simulink model "benchmark"  (R2019b)
settings: Solver=ode45  StartTime=0.0  StopTime=14  FixedStep=0.01  RelTol=1e-5  AbsTol=1e-8
values from neighbouring files (symbols this model uses):
  carb1 = 0    [asm1init.m]
  carb2 = 0    [asm1init.m]
  carb3 = 0    [asm1init.m]
  carb4 = 0    [asm1init.m]
  carb5 = 0    [asm1init.m]
  DIM = [ area height ]    [settler1dinit.m]
  Kfeedforward = 0    [reginit.m]
  KLa1 = 0    [asm1init.m]
  KLa2 = 0    [asm1init.m]
  KLa3 = 240    [asm1init.m]
  KLa4 = 240    [asm1init.m]
  KLa5_max = 360    [sensorinit.m]
  KLa5offset = 144    [reginit.m]
  KQintr = 10000    [reginit.m]
  KSO5 = 25    [reginit.m]
  LAYER = [ feedlayer nooflayers ]    [settler1dinit.m]
  max_SNO2 = 20    [sensorinit.m]
  max_SO5 = 10    [sensorinit.m]
  min_SNO2 = 0    [sensorinit.m]
  min_SO5 = 0    [sensorinit.m]
  MODELTYPE = [ 0 ]    [settler1dinit.m]
  noiseseed_SNO2 = 2    [sensorinit.m]
  noiseseed_SO5 = 1    [sensorinit.m]
  noisesource_SNO2 = 1    [sensorinit.m]
  noisesource_SO5 = 1    [sensorinit.m]
  PAR1 = [ mu_H  K_S  K_OH  K_NO  b_H  mu_A  K_NH  K_OA  b_A  ny_g  k_a  k_h  K_X  ny_h  Y_H  Y_A  f_P  i_XB  i_XP X_I2TSS  X_S2TSS  X_BH2TSS  X_BA2TSS  X_P2TSS ]    [asm1init.m]
  PAR2 = PAR1    [asm1init.m]
  PAR3 = PAR1    [asm1init.m]
  PAR4 = PAR1    [asm1init.m]
  PAR5 = PAR1    [asm1init.m]
  Qffref = 3    [reginit.m]
  Qin0 = 18446    [asm1init.m]    (also in states.mat)
  Qintr = 3*Qin0    (= 55338)    [asm1init.m]    (also in savestatesdyn.m = Qintrreg(:,3); states.mat = 16194.6247784)
  Qintr_max = 5*Qin0    [sensorinit.m]
  Qintrawstate = 0    [reginit.m]    (also in states.mat)
  Qintrintstate = 0    [reginit.m]    (also in states.mat = -1584.65140052)
  Qintroffset = 18500    [reginit.m]
  QintrT = T*10    (= 0.001)    [asm1init.m]
  SETTLERINIT = [ TSS_1 TSS_2 TSS_3 TSS_4 TSS_5 TSS_6 TSS_7 TSS_8 TSS_9 TSS_10  SI_1 SI_2 SI_3 SI_4 SI_5 SI_6 SI_7 SI_8 SI_9 SI_10  SS_1 SS_2 SS_3 SS_4 SS_5 SS_6 SS_7 SS_8 SS_9 SS_10  SO_1 SO_2 SO_3 SO_4 SO_5 SO_6 SO_7 SO_8 SO_9 SO_10  SNO_1 SNO_2 SNO_3 SNO_4 SNO_5 SNO_6 SNO_7 SNO_8 SNO_9 SNO_10  SNH_1 SNH_2 SNH_3 SNH_4 SNH_5 SNH_6 SNH_7 SNH_8 SNH_9 SNH_10 SND_1 SND_2 SND_3 SND_4 SND_5 SND_6 SND_7 SND_8 SND_9 SND ...(+77 chars)    [savestatesdyn.m]    (also in settler1dinit.m; states.mat = [12.59234379 18.2836278135 29.6255352805 68.5613149178 351.4)
  SETTLERPAR = [ v0_max v0 r_h r_p f_ns X_t ]    [settler1dinit.m]
  SNO2ref = 1    [reginit.m]
  SO5awstate = 0    [reginit.m]    (also in states.mat = 333.995683123)
  SO5intstate = 0    [reginit.m]    (also in states.mat = -324.385367613)
  SO5ref = 2    [reginit.m]
  SOSAT1 = 8    [asm1init.m]
  SOSAT2 = SOSAT1    (= 8)    [asm1init.m]
  SOSAT3 = SOSAT1    (= 8)    [asm1init.m]
  SOSAT4 = SOSAT1    (= 8)    [asm1init.m]
  SOSAT5 = SOSAT1    (= 8)    [asm1init.m]
  std_SNO2 = 0.025    [sensorinit.m]
  std_SO5 = 0.025    [sensorinit.m]
  T = 0.0001    [asm1init.m]
  T_KLa5 = T90_KLa5/(24*60)/3.89    (= 0.000714081690945)    [sensorinit.m]
  T_SNO2 = T90_SNO2/(24*60)/11.7724    (= 0.000589891988417)    [sensorinit.m]
  T_SO5 = T90_SO5/(24*60)/3.89    (= 0.000178520422736)    [sensorinit.m]
  TiQintr = 0.025    [reginit.m]
  TiSO5 = 0.002    [reginit.m]
  TtQintr = 0.015    [reginit.m]
  TtSO5 = 0.001    [reginit.m]
  useantiwindupQintr = 1    [reginit.m]
  useantiwindupSO5 = 1    [reginit.m]
  useideal_KLa5 = 0    [sensorinit.m]
  useideal_SNO2 = 0    [sensorinit.m]
  useideal_SO5 = 0    [sensorinit.m]
  usenoise_SNO2 = 1    [sensorinit.m]
  usenoise_SO5 = 1    [sensorinit.m]
  VOL1 = 1000    [asm1init.m]
  VOL2 = VOL1    (= 1000)    [asm1init.m]
  VOL3 = 1333    [asm1init.m]
  VOL4 = VOL3    (= 1333)    [asm1init.m]
  VOL5 = VOL3    (= 1333)    [asm1init.m]
  XINIT1 = XINIT1.*(rand(1, 15)/2)    [asm1init.m]    (also in savestatesdyn.m = [ S_I1  S_S1  X_I1  X_S1  X_BH1  X_BA1  X_P1  S_O1  S_NO1  S; states.mat = [30 3.19850453028 1132.76234619 97.3159244857 2519.85046875 )
  XINIT2 = XINIT2.*(rand(1, 15)/2)    [asm1init.m]    (also in savestatesdyn.m = [ S_I2  S_S2  X_I2  X_S2  X_BH2  X_BA2  X_P2  S_O2  S_NO2  S; states.mat = [30 1.66685060474 1124.48673742 89.8629588992 2501.10529682 )
  XINIT3 = XINIT3.*(rand(1, 15)/2)    [asm1init.m]    (also in savestatesdyn.m = [ S_I3  S_S3  X_I3  X_S3  X_BH3  X_BA3  X_P3  S_O3  S_NO3  S; states.mat = [30 1.21920729218 1120.83917563 67.9873482569 2499.89769316 )
  XINIT4 = XINIT4.*(rand(1, 15)/2)    [asm1init.m]    (also in savestatesdyn.m = [ S_I4  S_S4  X_I4  X_S4  X_BH4  X_BA4  X_P4  S_O4  S_NO4  S; states.mat = [30 0.970059599738 1121.87647389 52.9944958383 2504.40148464)
  XINIT5 = XINIT5.*(rand(1, 15)/2)    [asm1init.m]    (also in savestatesdyn.m = [ S_I5  S_S5  X_I5  X_S5  X_BH5  X_BA5  X_P5  S_O5  S_NO5  S; states.mat = [30 0.802872668211 1124.31099208 43.2311724286 2508.27851004)
  XINITDELAY = [ S_I_ASin  S_S_ASin  X_I_ASin  X_S_ASin  X_BH_ASin  X_BA_ASin  X_P_ASin  S_O_ASin  S_NO_ASin  S_NH_ASin  S_ND_ASin  X_ND_ASin  S_ALK_ASin TSS_ASin Q_ASin ]    [asm1init.m]    (also in savestatesdyn.m; states.mat = [1591648.02176 1269347.74818 60483506.753 5993584.75542 1336)
settings Model: ExtModeTrigMode=oneshot  ExtModeArmWhenConnect=off  ExtModeAutoUpdateStatusClock=off  Creator=ielulf  LastModifiedBy=ielsaagi
settings SolverCC: AutoScaleAbsTol=off
settings DataIOCC: SaveFormat=Array  SignalLoggingSaveFormat=ModelDataLogs  SaveOutput=off  ReturnWorkspaceOutputs=off  TimeSaveName=t  SignalLoggingName=sigsOut  OutputOption=SpecifiedOutputTimes  OutputTimes=[7:(1/96):14]
settings OptimizationCC: BlockReduction=off  BooleanDataType=off  InitFltsAndDblsToZero=on  LifeSpan=inf
settings DebuggingCC: AlgebraicLoopMsg=none  SaveWithParameterizedLinksMsg=none  UnderspecifiedInitializationDetection=Classic  MergeDetectMultiDrivingBlocksExec=none  SignalResolutionControl=TryResolveAllWithWarning  InheritedTsInSrcMsg=none  MultiTaskDSMMsg=warning  MultiTaskCondExecSysMsg=none  FcnCallInpInsideContextMsg=warning  UnconnectedOutputMsg=none  SFUnexpectedBacktrackingDiag=warning  SFNoUnconditionalDefaultTransitionDiag=warning  SFExecutionAtInitializationDiag=none  ArithmeticOperatorsInVariantConditions=warning
settings HardwareCC: ProdBitPerPointer=32  ProdBitPerSizeT=32  ProdBitPerPtrDiffT=32  ProdLargestAtomicFloat=None  ProdIntDivRoundTo=Undefined  ProdEndianess=Unspecified  ProdWordSize=32  ProdHWDeviceType=32-bit Generic  TargetUnknown=on
settings ModelReferenceCC: PropagateSignalLabelsOutOfModel=off
settings RTWCC: TemplateMakefile=grt_unix.tmf
settings CodeAppCC: StateflowObjectComments=on
settings GRTTargetCC: TargetFcnLib=ansi_tfl_tmw.mat  TargetLangStandard=C89/C90 (ANSI)  CombineOutputUpdateFcns=off  GRTInterface=on
settings ConfigComp: CovMetricSettings=dw  CovHtmlReporting=on  CovSaveCumulativeToWorkspaceVar=on  CovSaveSingleToWorkspaceVar=on

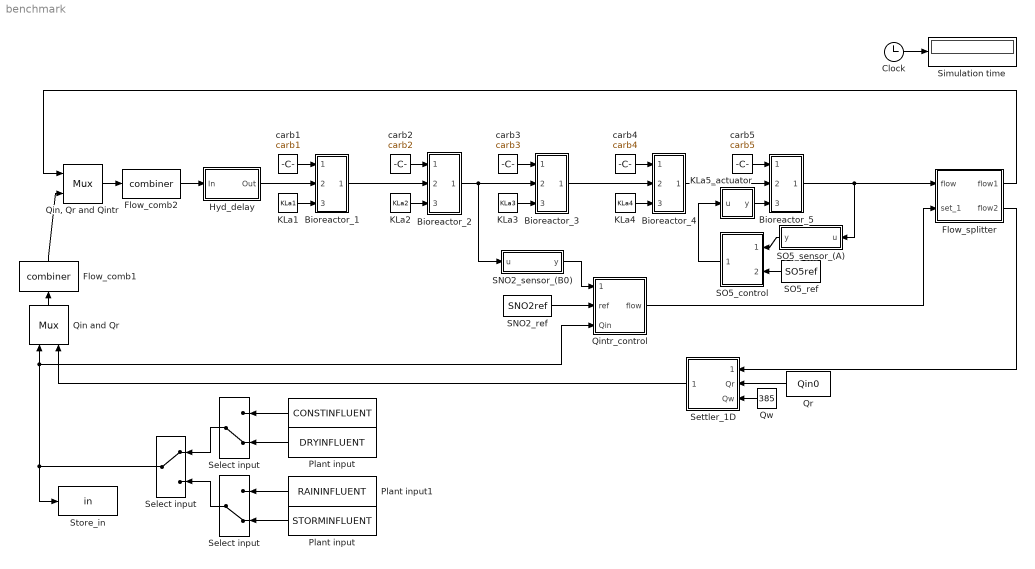
== system benchmark ==
  " " : FromWorkspace  VariableName=CONSTINFLUENT  OutputAfterFinalValue=Holding final value
  " Select input" : ManualSwitch
  Bioreactor_1 : Subsystem
  Bioreactor_2 : Subsystem
  Bioreactor_3 : Subsystem
  Bioreactor_4 : Subsystem
  Bioreactor_5 : Subsystem
  Clock : Clock
  Flow_comb1 : S-Function  FunctionName=combiner  SFunctionDeploymentMode=off  EnableBusSupport=off
  Flow_comb2 : S-Function  FunctionName=combiner  SFunctionDeploymentMode=off  EnableBusSupport=off
  Flow_splitter : Subsystem
  Hyd_delay : Subsystem
  KLa1 : Constant  Value=KLa1
  KLa2 : Constant  Value=KLa2
  KLa3 : Constant  Value=KLa3
  KLa4 : Constant  Value=KLa4
  KLa5_actuator : Subsystem
  Plant input : FromWorkspace  VariableName=DRYINFLUENT  OutputAfterFinalValue=Holding final value
  "Plant input " : FromWorkspace  VariableName=STORMINFLUENT  OutputAfterFinalValue=Holding final value
  Plant input1 : FromWorkspace  VariableName=RAININFLUENT  OutputAfterFinalValue=Holding final value
  Qin and Qr : Mux  Inputs=2
  "Qin, Qr and Qintr" : Mux  Inputs=2
  Qintr_control : Subsystem
  Qr : Constant  Value=Qin0
  Qw : Constant  Value=385
  SNO2_ref : Constant  Value=SNO2ref
  SNO2_sensor_(B0) : Subsystem
  SO5_control : Subsystem
  SO5_ref : Constant  Value=SO5ref
  SO5_sensor_(A) : Subsystem
  Select input : ManualSwitch  CurrentSetting=0
  "Select input " : ManualSwitch  CurrentSetting=0
  Settler_1D : Subsystem
  Simulation time : Display
  Store_in : ToWorkspace  VariableName=in  SampleTime=-1
  carb1 : Constant  Value=carb1
  carb2 : Constant  Value=carb2
  carb3 : Constant  Value=carb3
  carb4 : Constant  Value=carb4
  carb5 : Constant  Value=carb5
  wires:
  Qin and Qr/1 -> Flow_comb1/1
  Flow_comb1/1 -> "Qin, Qr and Qintr"/2
  "Qin, Qr and Qintr"/1 -> Flow_comb2/1
  Flow_splitter/1(flow1) -> "Qin, Qr and Qintr"/1
  Settler_1D/1(output) -> Qin and Qr/2
  Qw/1 -> Settler_1D/3(Qw)
  Flow_splitter/2(flow2) -> Settler_1D/1(feed)
  Qr/1 -> Settler_1D/2(Qr)
  Bioreactor_5/1(out) -> Flow_splitter/1(flow), SO5_sensor_(A)/1(u)
  Flow_comb2/1 -> Hyd_delay/1(In)
  Clock/1 -> Simulation time/1
  Plant input/1 -> Select input/2
  " "/1 -> Select input/1
  Hyd_delay/1(Out) -> Bioreactor_1/2(in)
  carb1/1 -> Bioreactor_1/1(carb)
  KLa1/1 -> Bioreactor_1/3(KLa)
  Bioreactor_1/1(out) -> Bioreactor_2/2(in)
  KLa2/1 -> Bioreactor_2/3(KLa)
  carb2/1 -> Bioreactor_2/1(carb)
  Bioreactor_2/1(out) -> Bioreactor_3/2(in), SNO2_sensor_(B0)/1(u)
  KLa3/1 -> Bioreactor_3/3(KLa)
  carb3/1 -> Bioreactor_3/1(carb)
  Bioreactor_3/1(out) -> Bioreactor_4/2(in)
  KLa4/1 -> Bioreactor_4/3(KLa)
  carb4/1 -> Bioreactor_4/1(carb)
  Bioreactor_4/1(out) -> Bioreactor_5/2(in)
  carb5/1 -> Bioreactor_5/1(carb)
  Plant input1/1 -> "Select input "/1
  "Plant input "/1 -> "Select input "/2
  Select input/1 -> " Select input"/1
  "Select input "/1 -> " Select input"/2
  " Select input"/1 -> Store_in/1, Qin and Qr/1, Qintr_control/3(Qin)
  SNO2_ref/1 -> Qintr_control/2(ref)
  SNO2_sensor_(B0)/1(y) -> Qintr_control/1(meas)
  Qintr_control/1(flow) -> Flow_splitter/2(set_1)
  SO5_ref/1 -> SO5_control/2(O2_ref)
  KLa5_actuator/1(y) -> Bioreactor_5/3(KLa)
  SO5_control/1(KLa) -> KLa5_actuator/1(u)
  SO5_sensor_(A)/1(y) -> SO5_control/1(O2_meas)

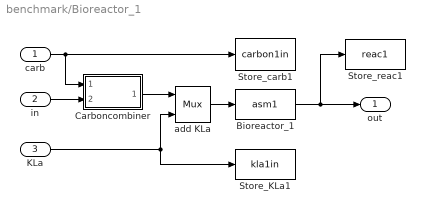
== system benchmark/Bioreactor_1 ==
  carb : Inport
  in : Inport  Port=2
  KLa : Inport  Port=3
  Bioreactor_1 : S-Function  FunctionName=asm1  Parameters=XINIT1,PAR1,VOL1,SOSAT1  SFunctionDeploymentMode=off  EnableBusSupport=off
  Carboncombiner : Subsystem
  Store_KLa1 : ToWorkspace  VariableName=kla1in  SampleTime=-1
  Store_carb1 : ToWorkspace  VariableName=carbon1in  SampleTime=-1
  Store_reac1 : ToWorkspace  VariableName=reac1  SampleTime=-1
  add KLa : Mux  Inputs=2
  out : Outport
  wires:
  add KLa/1 -> Bioreactor_1/1
  Bioreactor_1/1 -> out/1, Store_reac1/1
  Carboncombiner/1(Output) -> add KLa/1
  carb/1 -> Store_carb1/1, Carboncombiner/1(C_flow)
  in/1 -> Carboncombiner/2(Input)
  KLa/1 -> add KLa/2, Store_KLa1/1

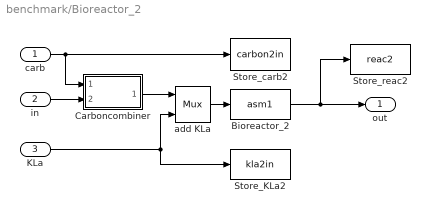
== system benchmark/Bioreactor_2 ==
  carb : Inport
  in : Inport  Port=2
  KLa : Inport  Port=3
  Bioreactor_2 : S-Function  FunctionName=asm1  Parameters=XINIT2,PAR2,VOL2,SOSAT2  SFunctionDeploymentMode=off  EnableBusSupport=off
  Carboncombiner : Subsystem
  Store_KLa2 : ToWorkspace  VariableName=kla2in  SampleTime=-1
  Store_carb2 : ToWorkspace  VariableName=carbon2in  SampleTime=-1
  Store_reac2 : ToWorkspace  VariableName=reac2  SampleTime=-1
  add KLa : Mux  Inputs=2
  out : Outport
  wires:
  Bioreactor_2/1 -> out/1, Store_reac2/1
  add KLa/1 -> Bioreactor_2/1
  Carboncombiner/1(Output) -> add KLa/1
  carb/1 -> Carboncombiner/1(C_flow), Store_carb2/1
  in/1 -> Carboncombiner/2(Input)
  KLa/1 -> add KLa/2, Store_KLa2/1

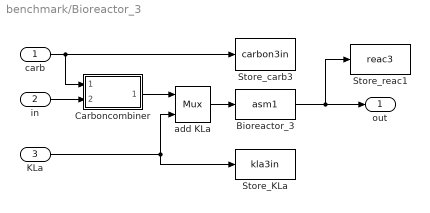
== system benchmark/Bioreactor_3 ==
  carb : Inport
  in : Inport  Port=2
  KLa : Inport  Port=3
  Bioreactor_3 : S-Function  FunctionName=asm1  Parameters=XINIT3,PAR3,VOL3,SOSAT3  SFunctionDeploymentMode=off  EnableBusSupport=off
  Carboncombiner : Subsystem
  Store_KLa : ToWorkspace  VariableName=kla3in  SampleTime=-1
  Store_carb3 : ToWorkspace  VariableName=carbon3in  SampleTime=-1
  Store_reac1 : ToWorkspace  VariableName=reac3  SampleTime=-1
  add KLa : Mux  Inputs=2
  out : Outport
  wires:
  Bioreactor_3/1 -> out/1, Store_reac1/1
  add KLa/1 -> Bioreactor_3/1
  Carboncombiner/1(Output) -> add KLa/1
  carb/1 -> Carboncombiner/1(C_flow), Store_carb3/1
  in/1 -> Carboncombiner/2(Input)
  KLa/1 -> add KLa/2, Store_KLa/1

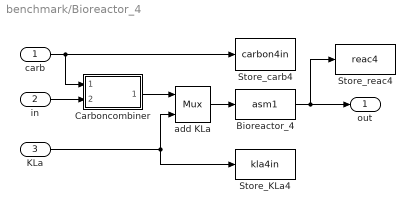
== system benchmark/Bioreactor_4 ==
  carb : Inport
  in : Inport  Port=2
  KLa : Inport  Port=3
  Bioreactor_4 : S-Function  FunctionName=asm1  Parameters=XINIT4,PAR4,VOL4,SOSAT4  SFunctionDeploymentMode=off  EnableBusSupport=off
  Carboncombiner : Subsystem
  Store_KLa4 : ToWorkspace  VariableName=kla4in  SampleTime=-1
  Store_carb4 : ToWorkspace  VariableName=carbon4in  SampleTime=-1
  Store_reac4 : ToWorkspace  VariableName=reac4  SampleTime=-1
  add KLa : Mux  Inputs=2
  out : Outport
  wires:
  Bioreactor_4/1 -> out/1, Store_reac4/1
  add KLa/1 -> Bioreactor_4/1
  Carboncombiner/1(Output) -> add KLa/1
  carb/1 -> Carboncombiner/1(C_flow), Store_carb4/1
  in/1 -> Carboncombiner/2(Input)
  KLa/1 -> add KLa/2, Store_KLa4/1

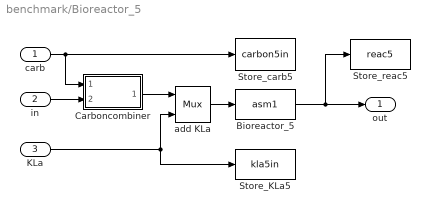
== system benchmark/Bioreactor_5 ==
  carb : Inport
  in : Inport  Port=2
  KLa : Inport  Port=3
  Bioreactor_5 : S-Function  FunctionName=asm1  Parameters=XINIT5,PAR5,VOL5,SOSAT5  SFunctionDeploymentMode=off  EnableBusSupport=off
  Carboncombiner : Subsystem
  Store_KLa5 : ToWorkspace  VariableName=kla5in  SampleTime=-1
  Store_carb5 : ToWorkspace  VariableName=carbon5in  SampleTime=-1
  Store_reac5 : ToWorkspace  VariableName=reac5  SampleTime=-1
  add KLa : Mux  Inputs=2
  out : Outport
  wires:
  Bioreactor_5/1 -> out/1, Store_reac5/1
  add KLa/1 -> Bioreactor_5/1
  Carboncombiner/1(Output) -> add KLa/1
  carb/1 -> Carboncombiner/1(C_flow), Store_carb5/1
  in/1 -> Carboncombiner/2(Input)
  KLa/1 -> add KLa/2, Store_KLa5/1

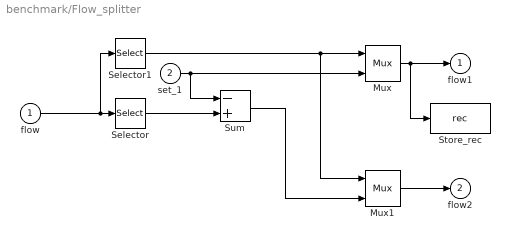
== system benchmark/Flow_splitter ==
  flow : Inport
  set_1 : Inport  Port=2
  Mux : Mux  Inputs=2
  Mux1 : Mux  Inputs=2
  Selector : Selector  InputPortWidth=15  IndexOptions=Index vector (dialog)  Indices=[15]  OutputSizes=1
  Selector1 : Selector  InputPortWidth=15  IndexOptions=Index vector (dialog)  Indices=[1 2 3 4 5 6 7 8 9 10 11 12 13 14]  OutputSizes=1
  Store_rec : ToWorkspace  VariableName=rec  SampleTime=-1
  Sum : Sum  Inputs=-+  SaturateOnIntegerOverflow=on  InputSameDT=on  OutDataTypeStr=Inherit: Same as first input
  flow1 : Outport
  flow2 : Outport  Port=2
  wires:
  flow/1 -> Selector1/1, Selector/1
  Mux/1 -> flow1/1, Store_rec/1
  Mux1/1 -> flow2/1
  set_1/1 -> Mux/2, Sum/1
  Selector/1 -> Sum/2
  Sum/1 -> Mux1/2
  Selector1/1 -> Mux/1, Mux1/1

== system benchmark/Hyd_delay ==
  In : Inport
  Demux : Demux  Outputs=[14,1]
  Hyd_delay : S-Function  FunctionName=hyddelayv3  Parameters=XINITDELAY,PAR1,T  SFunctionDeploymentMode=off  EnableBusSupport=off
  Mux : Mux  Inputs=2
  Product : Product  SaturateOnIntegerOverflow=on  OutDataTypeStr=Inherit: Same as first input
  Store_ASinput : ToWorkspace  VariableName=ASinput  SampleTime=-1
  Out : Outport
  wires:
  In/1 -> Hyd_delay/1
  Hyd_delay/1 -> Out/1, Demux/1
  Demux/1 -> Product/1
  Demux/2 -> Product/2, Mux/2
  Product/1 -> Mux/1
  Mux/1 -> Store_ASinput/1

== system benchmark/KLa5_actuator ==
  u : Inport
  Constant2 : Constant  Value=useideal_KLa5
  KLa5_actuator : TransferFcn  Denominator=[ T_KLa5*T_KLa5, 2*T_KLa5, 1]
  Switch1 : Switch  Threshold=0.5
  y : Outport
  wires:
  u/1 -> KLa5_actuator/1, Switch1/1
  Switch1/1 -> y/1
  KLa5_actuator/1 -> Switch1/3
  Constant2/1 -> Switch1/2

== system benchmark/Qintr_control ==
  meas : Inport
  ref : Inport  Port=2
  Qin : Inport  Port=3
  Selector : Selector  InputPortWidth=15  IndexOptions=Index vector (dialog)  Indices=[15]  OutputSizes=1
  Sum : Sum  Inputs=-+  SaturateOnIntegerOverflow=on  InputSameDT=on  OutDataTypeStr=Inherit: Same as first input
  cont_PI2 : Subsystem
  flow : Outport
  wires:
  meas/1 -> Sum/1
  Sum/1 -> cont_PI2/1(Error)
  cont_PI2/1(Out) -> flow/1
  Qin/1 -> Selector/1
  ref/1 -> Sum/2, cont_PI2/2(SNOref)
  Selector/1 -> cont_PI2/3(Qin)

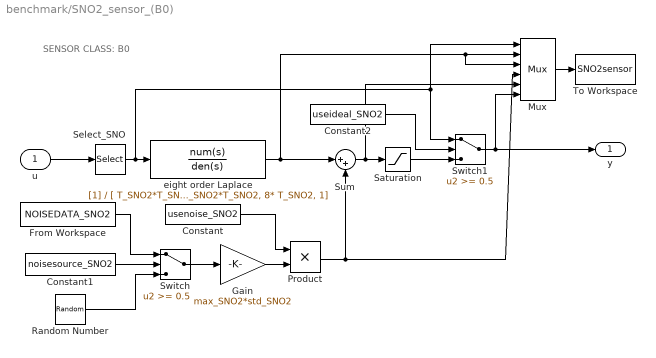
== system benchmark/SNO2_sensor_(B0) ==
  note: SENSOR CLASS: B0
  u : Inport
  Constant : Constant  Value=usenoise_SNO2
  Constant1 : Constant  Value=noisesource_SNO2
  Constant2 : Constant  Value=useideal_SNO2
  From Workspace : FromWorkspace  VariableName=NOISEDATA_SNO2  SampleTime=0
  Gain : Gain  Gain=max_SNO2*std_SNO2  SaturateOnIntegerOverflow=on  OutDataTypeStr=Inherit: Same as input  ParamDataTypeStr=Inherit: Same as input
  Mux : Mux  Inputs=6
  Product : Product  SaturateOnIntegerOverflow=on  InputSameDT=on  OutDataTypeStr=Inherit: Same as first input
  Random Number : RandomNumber  Seed=noiseseed_SNO2  SampleTime=1/1440
  Saturation : Saturate  UpperLimit=max_SNO2  LowerLimit=min_SNO2
  Select_SNO : Selector  InputPortWidth=15  IndexOptions=Index vector (dialog)  Indices=[9]  OutputSizes=1
  Sum : Sum  Inputs=|++  SaturateOnIntegerOverflow=on  InputSameDT=on  OutDataTypeStr=Inherit: Same as first input
  Switch : Switch  Threshold=0.5
  Switch1 : Switch  Threshold=0.5
  To Workspace : ToWorkspace  VariableName=SNO2sensor  SampleTime=-1
  eight order Laplace : TransferFcn  Denominator=[ T_SNO2*T_SNO2*T_SNO2*T_SNO2*T_SNO2*T_SNO2*T_SNO2*T_SNO2, 8*T_SNO2*T_SNO2*T_SNO2*T_SNO2*T_SNO2*T_SNO2*T_SNO2, 28*T_SNO2*T_SNO2*T_SNO2*T_SNO2*T_SNO2*T_SNO2, 56*T_SNO2*T_SNO2*T_SNO2*T_SNO2*T_SNO2, 70*T_SNO2*T_SNO2*T_SNO2*T_SNO2, 56*T_SNO2*T_SNO2*T_SNO2, 28*T_SNO2*T_SNO2, 8* T_SNO2, 1]
  y : Outport
  wires:
  Mux/1 -> To Workspace/1
  Constant2/1 -> Switch1/2
  Switch1/1 -> Mux/6, y/1
  Saturation/1 -> Switch1/3
  Random Number/1 -> Switch/3
  Constant1/1 -> Switch/2
  From Workspace/1 -> Switch/1
  Constant/1 -> Product/1
  Switch/1 -> Gain/1
  Gain/1 -> Product/2
  Select_SNO/1 -> Mux/1, Switch1/1, eight order Laplace/1
  u/1 -> Select_SNO/1
  Product/1 -> Mux/4, Sum/2
  eight order Laplace/1 -> Mux/3, Mux/2, Sum/1
  Sum/1 -> Mux/5, Saturation/1

== system benchmark/SO5_control ==
  O2_meas : Inport
  O2_ref : Inport  Port=2
  Sum : Sum  Inputs=-+  SaturateOnIntegerOverflow=on  InputSameDT=on  OutDataTypeStr=Inherit: Same as first input
  cont_PI : Subsystem
  KLa : Outport
  wires:
  Sum/1 -> cont_PI/1(In)
  O2_ref/1 -> Sum/2
  cont_PI/1(Out) -> KLa/1
  O2_meas/1 -> Sum/1

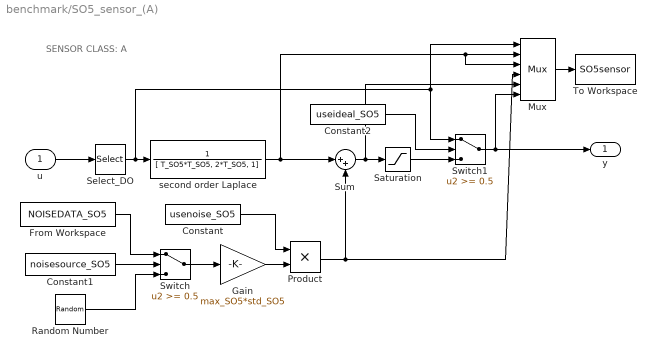
== system benchmark/SO5_sensor_(A) ==
  note: SENSOR CLASS: A
  u : Inport
  Constant : Constant  Value=usenoise_SO5
  Constant1 : Constant  Value=noisesource_SO5
  Constant2 : Constant  Value=useideal_SO5
  From Workspace : FromWorkspace  VariableName=NOISEDATA_SO5  SampleTime=0
  Gain : Gain  Gain=max_SO5*std_SO5  SaturateOnIntegerOverflow=on  OutDataTypeStr=Inherit: Same as input  ParamDataTypeStr=Inherit: Same as input
  Mux : Mux  Inputs=6
  Product : Product  SaturateOnIntegerOverflow=on  InputSameDT=on  OutDataTypeStr=Inherit: Same as first input
  Random Number : RandomNumber  Seed=noiseseed_SO5  SampleTime=1/1440
  Saturation : Saturate  UpperLimit=max_SO5  LowerLimit=min_SO5
  Select_DO : Selector  InputPortWidth=15  IndexOptions=Index vector (dialog)  Indices=[8]  OutputSizes=1
  Sum : Sum  Inputs=|++  SaturateOnIntegerOverflow=on  InputSameDT=on  OutDataTypeStr=Inherit: Same as first input
  Switch : Switch  Threshold=0.5
  Switch1 : Switch  Threshold=0.5
  To Workspace : ToWorkspace  VariableName=SO5sensor  SampleTime=-1
  second order Laplace : TransferFcn  Denominator=[ T_SO5*T_SO5, 2*T_SO5, 1]
  y : Outport
  wires:
  Mux/1 -> To Workspace/1
  Constant2/1 -> Switch1/2
  Switch1/1 -> Mux/6, y/1
  Saturation/1 -> Switch1/3
  Random Number/1 -> Switch/3
  Constant1/1 -> Switch/2
  From Workspace/1 -> Switch/1
  Constant/1 -> Product/1
  Switch/1 -> Gain/1
  Gain/1 -> Product/2
  Select_DO/1 -> Mux/1, Switch1/1, second order Laplace/1
  u/1 -> Select_DO/1
  Product/1 -> Mux/4, Sum/2
  second order Laplace/1 -> Mux/3, Mux/2, Sum/1
  Sum/1 -> Mux/5, Saturation/1

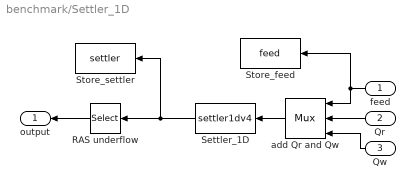
== system benchmark/Settler_1D ==
  feed : Inport
  Qr : Inport  Port=2
  Qw : Inport  Port=3
  RAS underflow : Selector  InputPortWidth=113  IndexOptions=Index vector (dialog)  Indices=[1 2 3 4 5 6 7 8 9 10 11 12 13 14 15]  OutputSizes=1
  Settler_1D : S-Function  FunctionName=settler1dv4  Parameters=SETTLERINIT,SETTLERPAR,DIM,LAYER,MODELTYPE  SFunctionDeploymentMode=off  EnableBusSupport=off
  Store_feed : ToWorkspace  VariableName=feed  SampleTime=-1
  Store_settler : ToWorkspace  VariableName=settler  SampleTime=-1
  add Qr and Qw : Mux  Inputs=3
  output : Outport
  wires:
  add Qr and Qw/1 -> Settler_1D/1
  Qr/1 -> add Qr and Qw/2
  Qw/1 -> add Qr and Qw/3
  feed/1 -> add Qr and Qw/1, Store_feed/1
  RAS underflow/1 -> output/1
  Settler_1D/1 -> RAS underflow/1, Store_settler/1

== system benchmark/Bioreactor_1/Carboncombiner ==
  C_flow : Inport
  Input : Inport  Port=2
  Carboncombiner : S-Function  FunctionName=carboncombiner  Parameters=CARBONSOURCECONC  SFunctionDeploymentMode=off  EnableBusSupport=off
  Mux : Mux  Inputs=2
  Output : Outport
  wires:
  C_flow/1 -> Mux/1
  Mux/1 -> Carboncombiner/1
  Carboncombiner/1 -> Output/1
  Input/1 -> Mux/2

== system benchmark/Bioreactor_2/Carboncombiner ==
  C_flow : Inport
  Input : Inport  Port=2
  Carboncombiner : S-Function  FunctionName=carboncombiner  Parameters=CARBONSOURCECONC  SFunctionDeploymentMode=off  EnableBusSupport=off
  Mux : Mux  Inputs=2
  Output : Outport
  wires:
  Input/1 -> Mux/2
  Carboncombiner/1 -> Output/1
  Mux/1 -> Carboncombiner/1
  C_flow/1 -> Mux/1

== system benchmark/Bioreactor_3/Carboncombiner ==
  C_flow : Inport
  Input : Inport  Port=2
  Carboncombiner : S-Function  FunctionName=carboncombiner  Parameters=CARBONSOURCECONC  SFunctionDeploymentMode=off  EnableBusSupport=off
  Mux : Mux  Inputs=2
  Output : Outport
  wires:
  Input/1 -> Mux/2
  Carboncombiner/1 -> Output/1
  Mux/1 -> Carboncombiner/1
  C_flow/1 -> Mux/1

== system benchmark/Bioreactor_4/Carboncombiner ==
  C_flow : Inport
  Input : Inport  Port=2
  Carboncombiner : S-Function  FunctionName=carboncombiner  Parameters=CARBONSOURCECONC  SFunctionDeploymentMode=off  EnableBusSupport=off
  Mux : Mux  Inputs=2
  Output : Outport
  wires:
  Input/1 -> Mux/2
  Carboncombiner/1 -> Output/1
  Mux/1 -> Carboncombiner/1
  C_flow/1 -> Mux/1

== system benchmark/Bioreactor_5/Carboncombiner ==
  C_flow : Inport
  Input : Inport  Port=2
  Carboncombiner : S-Function  FunctionName=carboncombiner  Parameters=CARBONSOURCECONC  SFunctionDeploymentMode=off  EnableBusSupport=off
  Mux : Mux  Inputs=2
  Output : Outport
  wires:
  Input/1 -> Mux/2
  Carboncombiner/1 -> Output/1
  Mux/1 -> Carboncombiner/1
  C_flow/1 -> Mux/1

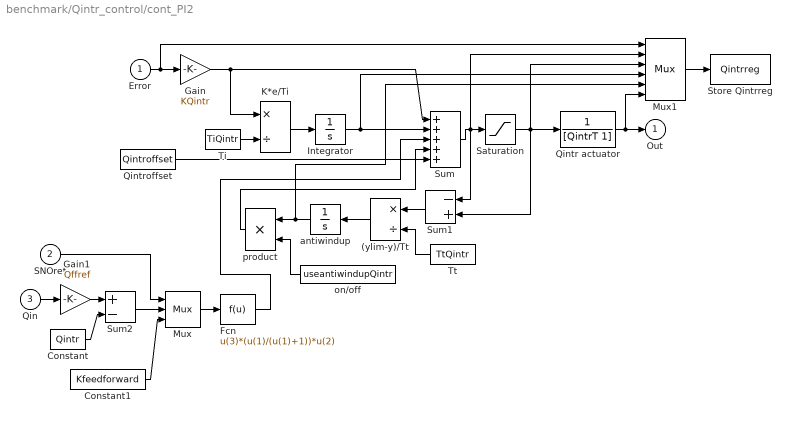
== system benchmark/Qintr_control/cont_PI2 ==
  Error : Inport
  SNOref : Inport  Port=2
  Qin : Inport  Port=3
  (ylim-y)/Tt : Product  Inputs=*/  SaturateOnIntegerOverflow=on  InputSameDT=on  OutDataTypeStr=Inherit: Same as first input
  Constant : Constant  Value=Qintr
  Constant1 : Constant  Value=Kfeedforward
  Fcn : Fcn  Expr=u(3)*(u(1)/(u(1)+1))*u(2)
  Gain : Gain  Gain=KQintr  SaturateOnIntegerOverflow=on  OutDataTypeStr=Inherit: Same as input  ParamDataTypeStr=Inherit: Same as input
  Gain1 : Gain  Gain=Qffref  SaturateOnIntegerOverflow=on  OutDataTypeStr=Inherit: Same as input  ParamDataTypeStr=Inherit: Same as input
  Integrator : Integrator  InitialCondition=Qintrintstate
  K*e/Ti : Product  Inputs=*/  SaturateOnIntegerOverflow=on  InputSameDT=on  OutDataTypeStr=Inherit: Same as first input
  Mux : Mux  Inputs=3
  Mux1 : Mux  Inputs=6
  Qintr actuator : TransferFcn  Denominator=[QintrT 1]
  Qintroffset : Constant  Value=Qintroffset
  Saturation : Saturate  UpperLimit=Qintr_max  LowerLimit=0
  Store Qintrreg : ToWorkspace  VariableName=Qintrreg  SampleTime=-1
  Sum : Sum  Inputs=+++++  SaturateOnIntegerOverflow=on  InputSameDT=on  OutDataTypeStr=Inherit: Same as first input
  Sum1 : Sum  Inputs=-+  SaturateOnIntegerOverflow=on  InputSameDT=on  OutDataTypeStr=Inherit: Same as first input
  Sum2 : Sum  Inputs=+-  SaturateOnIntegerOverflow=on  InputSameDT=on  OutDataTypeStr=Inherit: Same as first input
  Ti : Constant  Value=TiQintr
  Tt : Constant  Value=TtQintr
  antiwindup : Integrator  InitialCondition=Qintrawstate
  on/off : Constant  Value=useantiwindupQintr
  product : Product  Inputs=**  SaturateOnIntegerOverflow=on  InputSameDT=on  OutDataTypeStr=Inherit: Same as first input
  Out : Outport
  wires:
  Sum2/1 -> Mux/2
  Constant1/1 -> Mux/3
  on/off/1 -> product/2
  Error/1 -> Mux1/1, Gain/1
  Mux1/1 -> Store Qintrreg/1
  Saturation/1 -> Sum1/2, Qintr actuator/1, Mux1/3
  Sum/1 -> Mux1/2, Sum1/1, Saturation/1
  (ylim-y)/Tt/1 -> antiwindup/1
  Tt/1 -> (ylim-y)/Tt/2
  Sum1/1 -> (ylim-y)/Tt/1
  Gain/1 -> Sum/1, K*e/Ti/1
  Ti/1 -> K*e/Ti/2
  K*e/Ti/1 -> Integrator/1
  product/1 -> Sum/4
  SNOref/1 -> Mux/1
  Mux/1 -> Fcn/1
  Fcn/1 -> Sum/3
  Integrator/1 -> Sum/2, Mux1/4
  antiwindup/1 -> product/1, Mux1/5
  Constant/1 -> Sum2/2
  Qin/1 -> Gain1/1
  Gain1/1 -> Sum2/1
  Qintroffset/1 -> Sum/5
  Qintr actuator/1 -> Out/1, Mux1/6

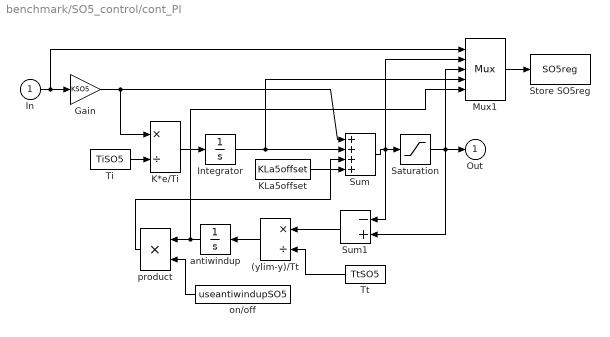
== system benchmark/SO5_control/cont_PI ==
  In : Inport
  (ylim-y)/Tt : Product  Inputs=*/  SaturateOnIntegerOverflow=on  InputSameDT=on  OutDataTypeStr=Inherit: Same as first input
  Gain : Gain  Gain=KSO5  SaturateOnIntegerOverflow=on  OutDataTypeStr=Inherit: Same as input  ParamDataTypeStr=Inherit: Same as input
  Integrator : Integrator  InitialCondition=SO5intstate
  K*e/Ti : Product  Inputs=*/  SaturateOnIntegerOverflow=on  InputSameDT=on  OutDataTypeStr=Inherit: Same as first input
  KLa5offset : Constant  Value=KLa5offset
  Mux1 : Mux  Inputs=5
  Saturation : Saturate  UpperLimit=KLa5_max  LowerLimit=0
  Store SO5reg : ToWorkspace  VariableName=SO5reg  SampleTime=-1
  Sum : Sum  Inputs=++++  SaturateOnIntegerOverflow=on  InputSameDT=on  OutDataTypeStr=Inherit: Same as first input
  Sum1 : Sum  Inputs=-+  SaturateOnIntegerOverflow=on  InputSameDT=on  OutDataTypeStr=Inherit: Same as first input
  Ti : Constant  Value=TiSO5
  Tt : Constant  Value=TtSO5
  antiwindup : Integrator  InitialCondition=SO5awstate
  on/off : Constant  Value=useantiwindupSO5
  product : Product  Inputs=**  SaturateOnIntegerOverflow=on  InputSameDT=on  OutDataTypeStr=Inherit: Same as first input
  Out : Outport
  wires:
  product/1 -> Sum/3
  on/off/1 -> product/2
  In/1 -> Mux1/1, Gain/1
  K*e/Ti/1 -> Integrator/1
  Ti/1 -> K*e/Ti/2
  Gain/1 -> Sum/1, K*e/Ti/1
  Sum1/1 -> (ylim-y)/Tt/1
  Tt/1 -> (ylim-y)/Tt/2
  (ylim-y)/Tt/1 -> antiwindup/1
  Sum/1 -> Saturation/1, Sum1/1, Mux1/2
  Saturation/1 -> Out/1, Sum1/2, Mux1/3
  Mux1/1 -> Store SO5reg/1
  Integrator/1 -> Sum/2, Mux1/4
  antiwindup/1 -> product/1, Mux1/5
  KLa5offset/1 -> Sum/4
